simulink model "oversamplingtest"  (R2014a)
settings: Solver=ode3  StartTime=0.0  StopTime=5.9  FixedStep=1/(16*2*pi)  RelTol=1e-3
libraries: dsparch4 x1
settings Model: Creator=Administratör  LastModifiedBy=Administratör

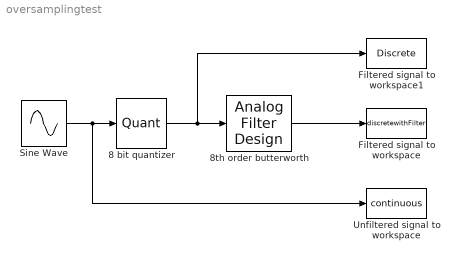
== system oversamplingtest ==
  8 bit quantizer : Quantizer  QuantizationInterval=2^-(2-1)
  8th order butterworth : dsparch4/Analog Filter Design  method=Butterworth  filttype=Lowpass  N=8  Wlo=2*2*pi  Whi=80  Rp=2  Rs=40
  Filtered signal to workspace : ToWorkspace  VariableName=discretewithFilter  SaveFormat=Structure With Time  SampleTime=-1
      settings: Decimation=4
  Filtered signal to workspace1 : ToWorkspace  VariableName=Discrete  SaveFormat=Structure With Time  SampleTime=-1
      settings: Decimation=4
  Sine Wave : Sin  Frequency=1*2*pi  SampleTime=0
  Unfiltered signal to workspace : ToWorkspace  VariableName=continuous  SaveFormat=Structure With Time  SampleTime=-1
      settings: Decimation=4
  wires:
  8 bit quantizer/1 -> Filtered signal to workspace1/1, 8th order butterworth/1
  Sine Wave/1 -> Unfiltered signal to workspace/1, 8 bit quantizer/1
  8th order butterworth/1 -> Filtered signal to workspace/1
